simulink model "OpenLoop_Test"  (R2023b)
settings: Solver=VariableStepAuto  StartTime=0.0  StopTime=10.0  RelTol=1e-3
libraries: cstblocks x6
settings Model: Creator=randolf  LastModifiedBy=randolf

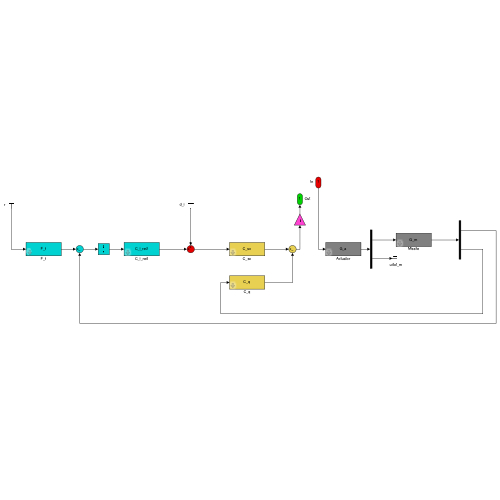
[thumbnail: Simulink's stored preview of the top-level diagram]
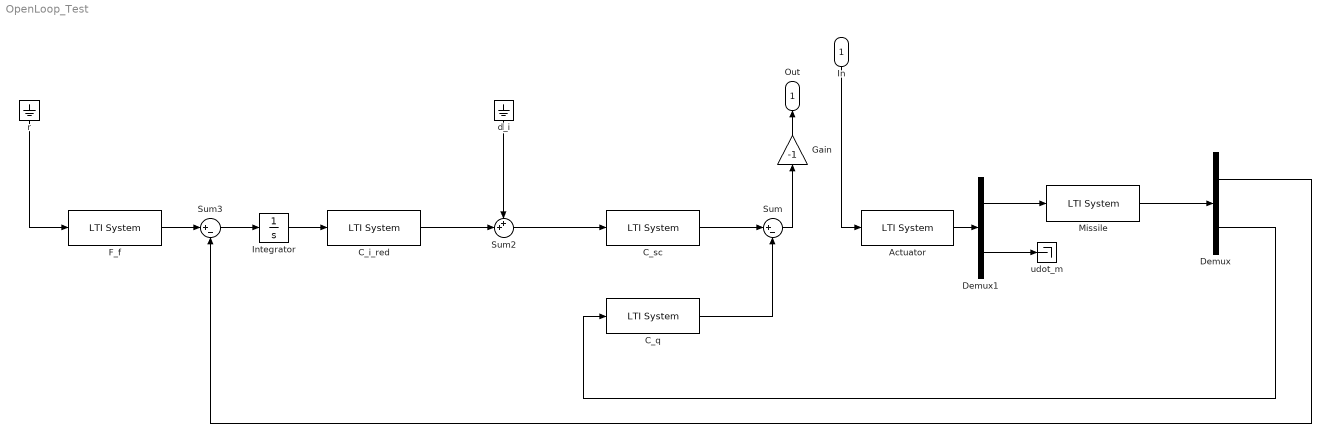
== system OpenLoop_Test ==
  In : Inport
  Actuator : cstblocks/LTI System  sys=G_a  IC=[]  PadeOrder=0
  C_i_red : cstblocks/LTI System  sys=C_i_red  IC=[]  PadeOrder=0
  C_q : cstblocks/LTI System  sys=C_q  IC=[]  PadeOrder=0
  C_sc : cstblocks/LTI System  sys=C_sc  IC=[]  PadeOrder=0
  Demux : Demux  Outputs=2
  Demux1 : Demux  Outputs=2
  F_f : cstblocks/LTI System  sys=F_f  IC=[]  PadeOrder=0
  Gain : Gain  Gain=-1
  Integrator : Integrator
  Missile : cstblocks/LTI System  sys=G_m  IC=[]  PadeOrder=0
  Sum : Sum  Inputs=|+-
  Sum2 : Sum  Inputs=++|
  Sum3 : Sum  Inputs=|+-
  d_i : Ground
  r : Ground
  udot_m : Terminator
  Out : Outport
  wires:
  Demux1/1 -> Missile/1
  C_i_red/1 -> Sum2/2
  Demux/2 -> C_q/1
  Actuator/1 -> Demux1/1
  Sum2/1 -> C_sc/1
  F_f/1 -> Sum3/1
  Sum3/1 -> Integrator/1
  Demux1/2 -> udot_m/1
  d_i/1 -> Sum2/1
  Missile/1 -> Demux/1
  Integrator/1 -> C_i_red/1
  C_q/1 -> Sum/2
  r/1 -> F_f/1
  C_sc/1 -> Sum/1
  Demux/1 -> Sum3/2
  Sum/1 -> Gain/1
  Gain/1 -> Out/1
  In/1 -> Actuator/1
